simulink model "Case1"  (R2021a)
settings: Solver=ode2  StartTime=0.0  StopTime=0.05  FixedStep=1000e-6  RelTol=1e-3
settings Model: Creator=s.ebrahimi  LastModifiedBy=s.ebrahimi
settings DebuggingCC: UnconnectedInputMsg=none  UnconnectedOutputMsg=none  UnconnectedLineMsg=none
settings ModelReferenceCC: EnableRefExpFcnMdlSchedulingChecks=off
settings RTWCC: Description=Generic Real-Time Target  GPUComputeCapability=5.0  DLArmComputeVersion=20.02.1

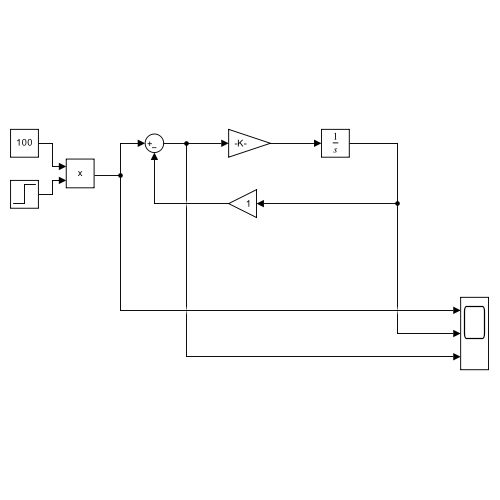
[thumbnail: Simulink's stored preview of the top-level diagram]
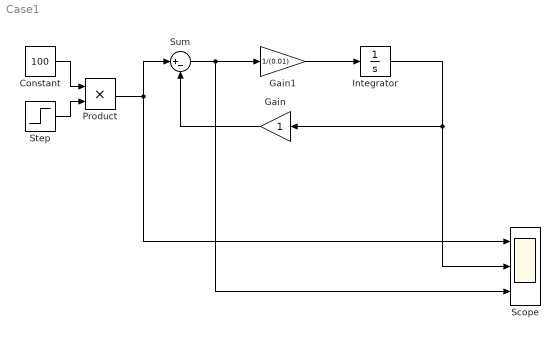
== system Case1 ==
  Constant : Constant  Value=100
  Gain : Gain
  Gain1 : Gain  Gain=1/(0.01)
  Integrator : Integrator
  Product : Product
  Scope : Scope  NumInputPorts=3
  Step : Step  Time=0.001  SampleTime=0
  Sum : Sum  Inputs=|+-
  wires:
  Constant/1 -> Product/1
  Gain/1 -> Sum/2
  Sum/1 -> Scope/3, Gain1/1
  Gain1/1 -> Integrator/1
  Integrator/1 -> Scope/2, Gain/1
  Step/1 -> Product/2
  Product/1 -> Scope/1, Sum/1
